simulink model "week1_5"  (R2020b)
settings: Solver=VariableStepAuto  StartTime=0.0  StopTime=10.0  RelTol=1e-3
PostLoadFcn:
  | clc;
  | clear all;
  | close all;
  | R=10;
  | C= 0.000001;
settings Model: Creator=hp  LastModifiedBy=hp

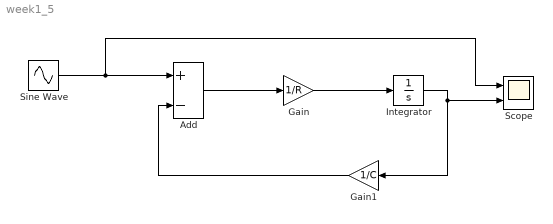
== system week1_5 ==
  Add : Sum  Inputs=+-
  Gain : Gain  Gain=1/R
  Gain1 : Gain  Gain=1/C
  Integrator : Integrator
  Scope : Scope  NumInputPorts=2
  Sine Wave : Sin  Amplitude=5  Frequency=3  SampleTime=0
  wires:
  Sine Wave/1 -> Scope/1, Add/1
  Add/1 -> Gain/1
  Gain1/1 -> Add/2
  Gain/1 -> Integrator/1
  Integrator/1 -> Gain1/1, Scope/2
